simulink model "hdlcoder_I2C_ssm2603"  (R2020b)
settings: Solver=FixedStepAuto  StartTime=0.0  StopTime=200000  FixedStep=1  MaxStep=1  MinStep=1  RelTol=1e-3
undefined symbols (not defined in the file or in its folder): I2C_Master_Controller, I2C_MasterController
settings Model: Creator=The MathWorks, Inc.  LastModifiedBy=amatsumo
settings SolverCC: InitialStep=1
settings DataIOCC: ReturnWorkspaceOutputs=off
settings OptimizationCC: BlockReduction=off  ConditionallyExecuteInputs=off  DefaultParameterBehavior=Inlined
settings DebuggingCC: AlgebraicLoopMsg=error  ArithmeticOperatorsInVariantConditions=warning
settings HardwareCC: ProdBitPerPointer=32  ProdBitPerSizeT=32  ProdBitPerPtrDiffT=32  ProdLargestAtomicFloat=None  ProdIntDivRoundTo=Undefined  ProdEndianess=Unspecified  ProdWordSize=32  ProdHWDeviceType=ASIC/FPGA->ASIC/FPGA  TargetBitPerPointer=64  TargetBitPerSizeT=64  TargetBitPerPtrDiffT=64  TargetLongLongMode=on  TargetIntDivRoundTo=Zero  TargetEndianess=LittleEndian  TargetWordSize=64  TargetHWDeviceType=MATLAB Host  ProdEqTarget=off
settings SFSimCC: SimUseLocalCustomCode=off  CustomCodeUndefinedFunction=UseInterfaceOnly
settings RTWCC: RTWUseLocalCustomCode=off
settings CodeAppCC: StateflowObjectComments=on

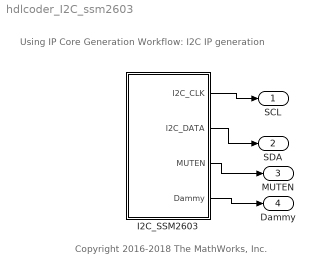
== system hdlcoder_I2C_ssm2603 ==
  note: Using IP Core Generation Workflow: I2C IP generation
  note: Copyright 2016-2018 The MathWorks, Inc.
  I2C_SSM2603 : Subsystem  TreatAsAtomicUnit=on
  SCL : Outport  VectorParamsAs1DForOutWhenUnconnected=off
  SDA : Outport  Port=2  VectorParamsAs1DForOutWhenUnconnected=off
  MUTEN : Outport  Port=3  VectorParamsAs1DForOutWhenUnconnected=off
  Dammy : Outport  Port=4  VectorParamsAs1DForOutWhenUnconnected=off
  wires:
  I2C_SSM2603/3(MUTEN) -> MUTEN/1
  I2C_SSM2603/1(I2C_CLK) -> SCL/1
  I2C_SSM2603/2(I2C_DATA) -> SDA/1
  I2C_SSM2603/4(Dammy) -> Dammy/1

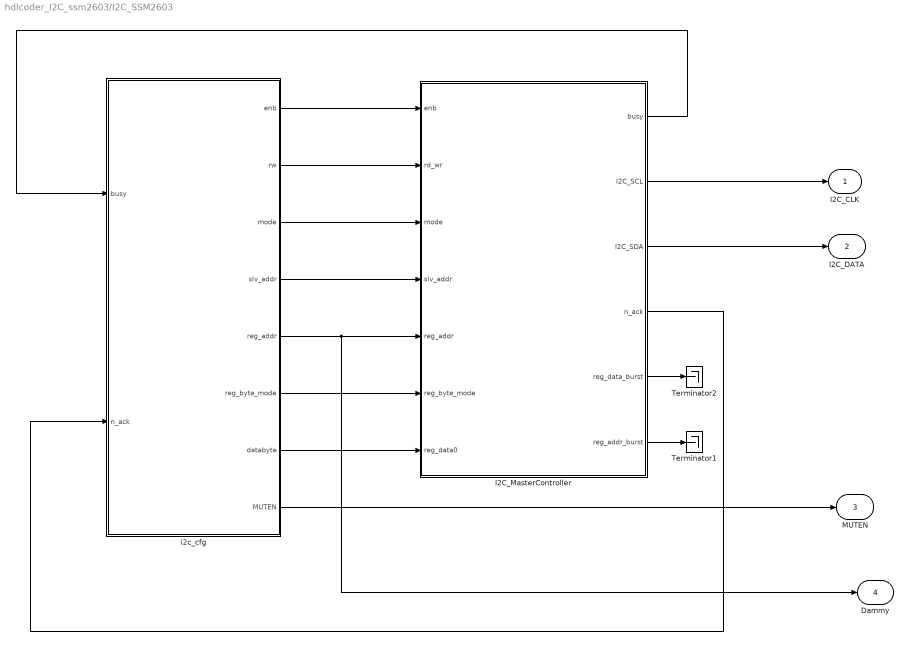
== system hdlcoder_I2C_ssm2603/I2C_SSM2603 ==
  I2C_MasterController : Subsystem  AncestorBlock=I2C_Master_Controller/I2C_MasterController
  Terminator1 : Terminator
  Terminator2 : Terminator
  i2c_cfg : Stateflow chart  TreatAsAtomicUnit=on
  I2C_CLK : Outport  VectorParamsAs1DForOutWhenUnconnected=off
  I2C_DATA : Outport  Port=2  VectorParamsAs1DForOutWhenUnconnected=off
  MUTEN : Outport  Port=3  VectorParamsAs1DForOutWhenUnconnected=off
  Dammy : Outport  Port=4  VectorParamsAs1DForOutWhenUnconnected=off
  wires:
  I2C_MasterController/2(I2C_SCL) -> I2C_CLK/1
  I2C_MasterController/3(I2C_SDA) -> I2C_DATA/1
  I2C_MasterController/1(busy) -> i2c_cfg/1(busy)
  I2C_MasterController/4(n_ack) -> i2c_cfg/2(n_ack)
  i2c_cfg/1(enb) -> I2C_MasterController/1(enb)
  i2c_cfg/2(rw) -> I2C_MasterController/2(rd_wr)
  i2c_cfg/3(mode) -> I2C_MasterController/3(mode)
  i2c_cfg/4(slv_addr) -> I2C_MasterController/4(slv_addr)
  i2c_cfg/5(reg_addr) -> Dammy/1, I2C_MasterController/5(reg_addr)
  i2c_cfg/6(reg_byte_mode) -> I2C_MasterController/6(reg_byte_mode)
  i2c_cfg/7(databyte) -> I2C_MasterController/7(reg_data0)
  i2c_cfg/8(MUTEN) -> MUTEN/1
  I2C_MasterController/5(reg_data_burst) -> Terminator2/1
  I2C_MasterController/6(reg_addr_burst) -> Terminator1/1

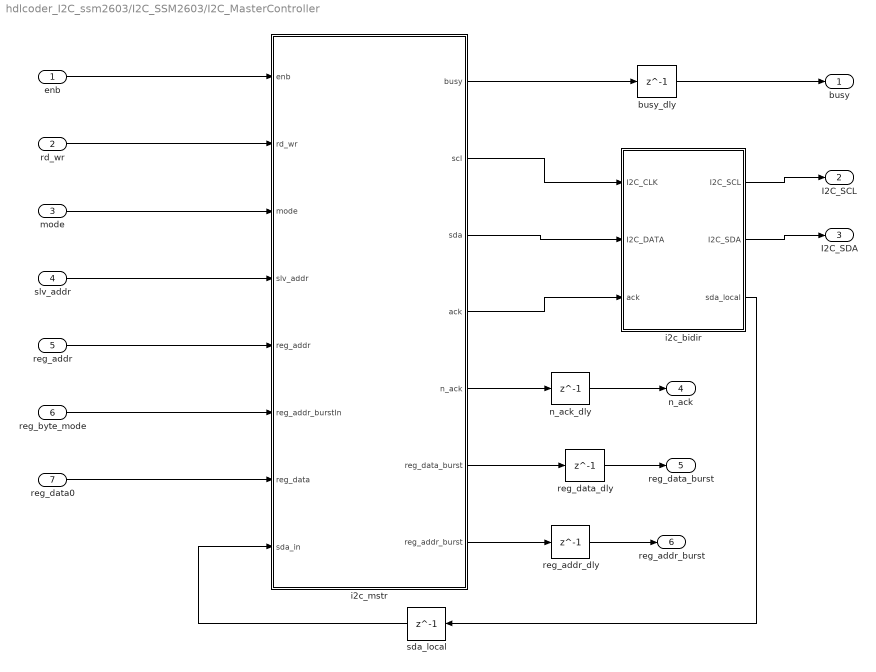
== system hdlcoder_I2C_ssm2603/I2C_SSM2603/I2C_MasterController ==
  enb : Inport
  rd_wr : Inport  Port=2
  mode : Inport  Port=3
  slv_addr : Inport  Port=4
  reg_addr : Inport  Port=5
  reg_byte_mode : Inport  Port=6
  reg_data0 : Inport  Port=7
  busy_dly : Delay  DelayLength=1
  i2c_bidir : Subsystem  TreatAsAtomicUnit=on
  i2c_mstr : Stateflow chart  TreatAsAtomicUnit=on
  n_ack_dly : Delay  DelayLength=1
  reg_addr_dly : Delay  DelayLength=1
  reg_data_dly : Delay  DelayLength=1
  sda_local : Delay  DelayLength=1
  busy : Outport  VectorParamsAs1DForOutWhenUnconnected=off
  I2C_SCL : Outport  Port=2  VectorParamsAs1DForOutWhenUnconnected=off
  I2C_SDA : Outport  Port=3  VectorParamsAs1DForOutWhenUnconnected=off
  n_ack : Outport  Port=4  VectorParamsAs1DForOutWhenUnconnected=off
  reg_data_burst : Outport  Port=5  VectorParamsAs1DForOutWhenUnconnected=off
  reg_addr_burst : Outport  Port=6  VectorParamsAs1DForOutWhenUnconnected=off
  wires:
  rd_wr/1 -> i2c_mstr/2(rd_wr)
  i2c_mstr/1(busy) -> busy_dly/1
  mode/1 -> i2c_mstr/3(mode)
  reg_data0/1 -> i2c_mstr/7(reg_data)
  i2c_mstr/7(reg_addr_burst) -> reg_addr_dly/1
  enb/1 -> i2c_mstr/1(enb)
  slv_addr/1 -> i2c_mstr/4(slv_addr)
  i2c_mstr/6(reg_data_burst) -> reg_data_dly/1
  reg_byte_mode/1 -> i2c_mstr/6(reg_addr_burstIn)
  reg_addr/1 -> i2c_mstr/5(reg_addr)
  sda_local/1 -> i2c_mstr/8(sda_in)
  i2c_mstr/5(n_ack) -> n_ack_dly/1
  reg_addr_dly/1 -> reg_addr_burst/1
  busy_dly/1 -> busy/1
  reg_data_dly/1 -> reg_data_burst/1
  n_ack_dly/1 -> n_ack/1
  i2c_mstr/2(scl) -> i2c_bidir/1(I2C_CLK)
  i2c_mstr/3(sda) -> i2c_bidir/2(I2C_DATA)
  i2c_mstr/4(ack) -> i2c_bidir/3(ack)
  i2c_bidir/1("I2C_SCL ") -> I2C_SCL/1
  i2c_bidir/2(I2C_SDA) -> I2C_SDA/1
  i2c_bidir/3(sda_local) -> sda_local/1

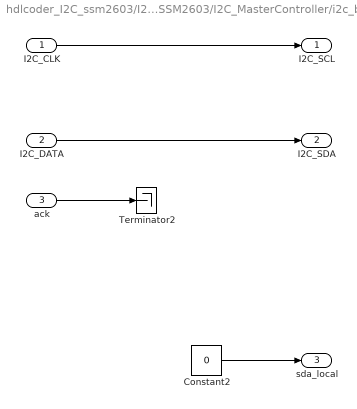
== system hdlcoder_I2C_ssm2603/I2C_SSM2603/I2C_MasterController/i2c_bidir ==
  I2C_CLK : Inport  OutDataTypeStr=boolean
  I2C_DATA : Inport  Port=2  OutDataTypeStr=boolean
  ack : Inport  Port=3  OutDataTypeStr=boolean
  Constant2 : Constant  Value=0  OutDataTypeStr=boolean  SampleTime=-1
  Terminator2 : Terminator
  "I2C_SCL " : Outport  OutDataTypeStr=boolean  VectorParamsAs1DForOutWhenUnconnected=off
  I2C_SDA : Outport  Port=2  OutDataTypeStr=boolean  VectorParamsAs1DForOutWhenUnconnected=off
  sda_local : Outport  Port=3  OutDataTypeStr=boolean  VectorParamsAs1DForOutWhenUnconnected=off
  wires:
  ack/1 -> Terminator2/1
  Constant2/1 -> sda_local/1
  I2C_DATA/1 -> I2C_SDA/1
  I2C_CLK/1 -> "I2C_SCL "/1

== stateflow chart hdlcoder_I2C_ssm2603/I2C_SSM2603/I2C_MasterController/i2c_mstr ==
  settings: executeAtInitialization=1
  note: I2C Master Controller
  state idle
    entry:
    scl(:) = 1
    sda(:) = 1
    busy(:)  = 0
  state stop_ext
    entry:
    scl (:) = 1
    sda(:) = 1
    ack(:) = 0
  state ready
    entry:
    scl(:) = 1
    sda(:) = 1
  state stop
    entry:
    sda(:) = 0
  state start_n
    entry:
    scl(:) = 1
    sda(:) = 0
    bit_cnt = 7
    busy(:) = 1
    reg_byte_cnt =1
  state scl_ext_p
    entry:
    scl(:) = 1
    sda(:) = 0
    ack(:) = 0
  state scl_ext_n
    entry:
    scl(:) = 0
    sda(:) = 0
    ack(:) = 0
  state start_p
    entry:
    sda(:) = 0
  state cmd_slave_addr_n
    entry:
    scl(:) = 0
    sda(:) = bitget(slv_addr,bit_cnt)
  state ack_data_cnf
    entry:
    scl(:) = 1
    ack (:) = 1
  state nack_data_cnf
    entry:
    scl(:) = 1
    n_ack (:) = 1
  state cmd_slave_addr_p
    entry:
    scl(:) = 1
    bit_cnt = bit_cnt-1
  state Increment_Byte_count
    entry:
    scl(:) = 1
    bit_cnt = 8
    ack (:) = 1
    reg_data_burst(:) = 1
  state Increment_Byte_count1
    entry:
    scl(:) = 1
    bit_cnt = 8
    n_ack (:) = 1
  state ack_data
    entry:
    scl(:) = 0
    sda(:) = 1
    ack(:) = 1
  state nack_data
    entry:
    scl(:) = 0
    sda(:) = 1
    n_ack(:) = 1
  state write_n
    entry:
    scl(:) = 0
    sda(:) = 0
  state read_state [commented out]
    entry:
    scl(:) = 0
    sda(:) = 1
  state cmd_reg_data_p
    entry:
    scl(:) = 1
    bit_cnt = bit_cnt-1
  state write_p
    entry:
    scl(:) = 1
    sda(:) = 0
  state cmd_reg_data_n
    entry:
    scl(:) = 0
    sda(:) = bitget(reg_data,bit_cnt);
    ack(:) = 0
    reg_data_burst(:) = 0
  state ack_slv
    entry:
    scl(:) = 0
    ack(:) = 1
    sda(:) = 1
  state nack_slv
    entry:
    scl(:) = 0
    sda(:) = 1
    n_ack(:) = 1
  state ack_slv_cnf
    entry:
    scl(:)= 1
    ack(:) = 1
    bit_cnt = 8
  state nack_slv_cnf
    entry:
    scl(:) =1
    bit_cnt = 8
    n_ack(:) = 1
  state nack_addrm1
    entry:
    scl(:) = 1
    n_ack(:) = 1
    bit_cnt = 8;
    %reg_mode(:)=1
  state cmd_reg_addr_n
    entry:
    scl(:) = 0
    ack(:) = 0
    sda(:) = bitget(reg_addr,bit_cnt);
    reg_addr_burst(:)=0
  state nack_addrm_cnf
    entry:
    scl(:) =1
    bit_cnt = 8;
    n_ack(:) = 1
  state nack_addrm
    entry:
    scl(:) = 0
    sda(:) = 1
    n_ack(:) = 1
  state cmd_reg_addr_p
    entry:
    scl(:)= 1
    bit_cnt = bit_cnt-1
  state ack_addr_m
    entry:
    scl(:) = 0
    ack (:) = 1
    sda(:) = 1
  state ack_addr_m_cnf
    entry:
    scl(:) = 1
    bit_cnt = 8;
    ack(:) = 1
  state ack_addrm1
    entry:
    scl(:) = 1
    ack(:) = 1
    bit_cnt = 8;
    reg_addr_burst(:)=1
  (default) -> idle
  stop_ext -> idle
  idle -> ready : [enb==1]
  stop -> stop_ext
  ready -> start_n
  scl_ext_p -> stop
  scl_ext_n -> scl_ext_p
  start_n -> start_p
  nack_data_cnf -> scl_ext_n
  ack_data_cnf -> scl_ext_n
  start_p -> cmd_slave_addr_n
  cmd_slave_addr_p -> cmd_slave_addr_n [order 1] : [bit_cnt > 0]
  cmd_slave_addr_n -> cmd_slave_addr_p
  ack_data -> ack_data_cnf [order 2]
  nack_data -> nack_data_cnf [order 2]
  cmd_slave_addr_p -> read_state [commented out] : [rd_wr==1]
  ack_data -> Increment_Byte_count [order 1] : [mode == 1]
  Increment_Byte_count -> cmd_reg_data_n
  nack_data -> Increment_Byte_count1 [order 1] : [mode == 1]
  cmd_slave_addr_p -> write_n [order 2] : [rd_wr== 0]
  cmd_reg_data_p -> nack_data [order 3]
  cmd_reg_data_p -> ack_data [order 2] : [sda_in == 0]
  Increment_Byte_count1 -> cmd_reg_data_n
  write_n -> write_p
  cmd_reg_data_p -> cmd_reg_data_n [order 1] : [bit_cnt > 0]
  cmd_reg_data_n -> cmd_reg_data_p
  write_p -> nack_slv [order 2]
  write_p -> ack_slv [order 1] : [sda_in == 0]
  ack_addr_m_cnf -> cmd_reg_data_n
  nack_addrm_cnf -> cmd_reg_data_n
  ack_slv -> ack_slv_cnf
  nack_slv -> nack_slv_cnf
  nack_slv_cnf -> cmd_reg_addr_n
  ack_slv_cnf -> cmd_reg_addr_n
  nack_addrm1 -> cmd_reg_addr_n
  ack_addrm1 -> cmd_reg_addr_n
  nack_addrm -> nack_addrm1 [order 1] : [reg_addr_burstIn ==1]
  cmd_reg_addr_p -> cmd_reg_addr_n [order 1] : [bit_cnt > 0]
  cmd_reg_addr_n -> cmd_reg_addr_p
  cmd_reg_addr_p -> nack_addrm [order 3]
  nack_addrm -> nack_addrm_cnf [order 2]
  cmd_reg_addr_p -> ack_addr_m [order 2] : [sda_in == 0]
  ack_addr_m -> ack_addr_m_cnf [order 2]
  ack_addr_m -> ack_addrm1 [order 1] : [reg_addr_burstIn ==1]
  data: enb input boolean size=1; rd_wr input boolean size=1; mode input boolean size=1; busy output boolean size=1; bit_cnt local uint8; scl output boolean size=1; sda output boolean size=1; slv_addr input uint8; reg_addr input uint8; reg_addr_burstIn input boolean size=1; reg_data input uint8; sda_in input boolean size=1; ack output boolean size=1; n_ack output boolean size=1; reg_byte_cnt local uint8; reg_data_burst output boolean size=1; reg_addr_burst output boolean size=1

== stateflow chart hdlcoder_I2C_ssm2603/I2C_SSM2603/i2c_cfg ==
  settings: executeAtInitialization=1
  note: I2C Configuration for SSM2603
  state init
    %initstate
    entry: enb 	= 0
    rw 		= 0
    mode 	= 0
    inc_in  = 0
    wait 	= 0
    %byte_mode = 0
    %reg_mode  = 0
    MUTEN =1
  state load_lut_data
    % Load lut data
    entry: enb 				  = 1
    rw  				  = 0
    reg_byte_mode 	  = 0
    slv_addr 	 	        = 0x1A
    reg_addr 	  =  reg_addr(inc_in);
    databyte 	  =  reg_data(inc_in);
  state y1  = reg_addr(lut_index) [function]
    (default) -> (junction 2155) : % load lut data
    (junction 2155) -> (junction 2156) [order 1] : [lut_index == 0]
    (junction 2156) -> (junction 2157) : {y1=0x0C;}
    (junction 2155) -> (junction 2159) [order 2]
    (junction 2157) -> (junction 2158)
    (junction 2158) -> (junction 2162)
    (junction 2159) -> (junction 2160) [order 1] : [lut_index == 1]
    (junction 2159) -> (junction 2163) [order 2]
    (junction 2160) -> (junction 2161) : {y1=0x00;}
    (junction 2161) -> (junction 2162)
    (junction 2162) -> (junction 2166)
    (junction 2163) -> (junction 2164) [order 1] : [lut_index == 2]
    (junction 2164) -> (junction 2165) : {y1=0x02;}
    (junction 2163) -> (junction 2167) [order 2]
    (junction 2165) -> (junction 2166)
    (junction 2166) -> (junction 2170)
    (junction 2167) -> (junction 2168) [order 1] : [lut_index == 3]
    (junction 2168) -> (junction 2169) : {y1=0x04;}
    (junction 2167) -> (junction 2171) [order 2]
    (junction 2169) -> (junction 2170)
    (junction 2170) -> (junction 2174)
    (junction 2171) -> (junction 2172) [order 1] : [lut_index == 4]
    (junction 2171) -> (junction 2175) [order 2]
    (junction 2172) -> (junction 2173) : {y1=0x06;}
    (junction 2173) -> (junction 2174)
    (junction 2174) -> (junction 2178)
    (junction 2175) -> (junction 2176) [order 1] : [lut_index == 5]
    (junction 2176) -> (junction 2177) : {y1=0x08;}
    (junction 2175) -> (junction 2179) [order 2]
    (junction 2177) -> (junction 2178)
    (junction 2178) -> (junction 2182)
    (junction 2179) -> (junction 2180) [order 1] : [lut_index == 6]
    (junction 2179) -> (junction 2183) [order 2]
    (junction 2180) -> (junction 2181) : {y1=0x0A;}
    (junction 2181) -> (junction 2182)
    (junction 2182) -> (junction 2186)
    (junction 2183) -> (junction 2184) [order 1] : [lut_index == 7]
    (junction 2184) -> (junction 2185) : {y1=0x0E;}
    (junction 2183) -> (junction 2187) [order 2]
    (junction 2185) -> (junction 2186)
    (junction 2186) -> (junction 2190)
    (junction 2187) -> (junction 2188) [order 1] : [lut_index == 8]
    (junction 2187) -> (junction 2191) [order 2]
    (junction 2188) -> (junction 2189) : {y1=0x10;}
    (junction 2189) -> (junction 2190)
    (junction 2190) -> (junction 2194)
    (junction 2191) -> (junction 2192) [order 1] : [lut_index == 9]
    (junction 2191) -> (junction 2195) [order 2] : {y1=0x00;}
    (junction 2192) -> (junction 2193) : {y1=0x0C;}
    (junction 2193) -> (junction 2194)
    (junction 2194) -> (junction 2196)
    (junction 2196) -> (junction 2195)
    (junction 2195) -> (junction 2197)
  state lut_incr1
    entry: inc_in++;
  state y3  = reg_data(lut_index) [function]
    (default) -> (junction 2256) : % load lut data
    (junction 2256) -> (junction 2257) [order 1] : [lut_index == 0]
    (junction 2257) -> (junction 2258) : {y3=0x10;}
    (junction 2256) -> (junction 2260) [order 2]
    (junction 2258) -> (junction 2259)
    (junction 2259) -> (junction 2263)
    (junction 2260) -> (junction 2261) [order 1] : [lut_index == 1]
    (junction 2260) -> (junction 2264) [order 2]
    (junction 2261) -> (junction 2262) : {y3=0x17;}
    (junction 2262) -> (junction 2263)
    (junction 2263) -> (junction 2267)
    (junction 2264) -> (junction 2265) [order 1] : [lut_index == 2]
    (junction 2265) -> (junction 2266) : {y3=0x17;}
    (junction 2264) -> (junction 2268) [order 2]
    (junction 2266) -> (junction 2267)
    (junction 2267) -> (junction 2271)
    (junction 2268) -> (junction 2269) [order 1] : [lut_index == 3]
    (junction 2269) -> (junction 2270) : {y3=0x79;}
    (junction 2268) -> (junction 2272) [order 2]
    (junction 2270) -> (junction 2271)
    (junction 2271) -> (junction 2275)
    (junction 2272) -> (junction 2273) [order 1] : [lut_index == 4]
    (junction 2272) -> (junction 2276) [order 2]
    (junction 2273) -> (junction 2274) : {y3=0x79;}
    (junction 2274) -> (junction 2275)
    (junction 2275) -> (junction 2279)
    (junction 2276) -> (junction 2277) [order 1] : [lut_index == 5]
    (junction 2277) -> (junction 2278) : {y3=0x12;}
    (junction 2276) -> (junction 2280) [order 2]
    (junction 2278) -> (junction 2279)
    (junction 2279) -> (junction 2283)
    (junction 2280) -> (junction 2281) [order 1] : [lut_index == 6]
    (junction 2280) -> (junction 2284) [order 2]
    (junction 2281) -> (junction 2282) : {y3=0x06;}
    (junction 2282) -> (junction 2283)
    (junction 2283) -> (junction 2287)
    (junction 2284) -> (junction 2285) [order 1] : [lut_index == 7]
    (junction 2285) -> (junction 2286) : {y3=0x4A;}
    (junction 2284) -> (junction 2288) [order 2]
    (junction 2286) -> (junction 2287)
    (junction 2287) -> (junction 2291)
    (junction 2288) -> (junction 2289) [order 1] : [lut_index == 8]
    (junction 2288) -> (junction 2292) [order 2]
    (junction 2289) -> (junction 2290) : {y3=0x20;}
    (junction 2290) -> (junction 2291)
    (junction 2291) -> (junction 2295)
    (junction 2292) -> (junction 2293) [order 1] : [lut_index == 9]
    (junction 2292) -> (junction 2296) [order 2] : {y3=0x00;}
    (junction 2293) -> (junction 2294) : {y3=0x00;}
    (junction 2294) -> (junction 2295)
    (junction 2295) -> (junction 2297)
    (junction 2297) -> (junction 2296)
    (junction 2296) -> (junction 2298)
  state finish1
    entry: enb = 0
  state wait_state1
    entry: wait = wait+1;
  state load_last_reg
    %Load last register
    entry: enb 	= 1
    rw 		= 0
    mode 	= 0
    slv_addr     = 0x1A
    reg_byte_mode = 0
    reg_addr 	  =  0x12
    databyte     = 0x01
  state end_state
    entry: enb 	 = 0
  (default) -> init
  init -> load_lut_data : [busy==0]
  lut_incr1 -> load_lut_data [order 1] : [inc_in < 10 & busy==0 ]
  load_lut_data -> lut_incr1 : [busy==0 & n_ack ==0]
  lut_incr1 -> finish1 [order 2] : [inc_in == 10]
  wait_state1 -> finish1 [order 2] : [busy == 0 & n_ack == 0 & wait != 800000]
  finish1 -> wait_state1 : [busy == 0 & n_ack==0]
  wait_state1 -> load_last_reg [order 1] : [busy==0 & n_ack ==0 & wait== 800000]
  load_last_reg -> end_state : [enb == 1]
  data: lut_index function_input double; y1 function_output double; lut_index function_input double; y3 function_output double; enb output boolean size=1; rw output boolean size=1; mode output boolean size=1; slv_addr output uint8; reg_addr output uint8; reg_byte_mode output boolean size=1; busy input; inc_in local uint8; databyte output uint8; n_ack input; wait local uint32; MUTEN output boolean size=1
